simulink model "quadrotor_model_simulink_validation"  (R2018a)
settings: Solver=FixedStepDiscrete  StartTime=0.0  StopTime=40  FixedStep=Ts  RelTol=1e-3
PreLoadFcn:
  | % Quadrotor model
  | load('quadrotor_model.mat');
  | Ts = quadrotor_model.Ts;
  | d = 3;
InitFcn:
  | % Quadrotor model
  | load('quadrotor_model.mat');
  | Ts = quadrotor_model.Ts;
  | d = 3;
undefined symbols (not defined in the file): quadrotor_model
settings Model: Creator=silveira  LastModifiedBy=silveira
settings DebuggingCC: ReadBeforeWriteMsg=DisableAll  WriteAfterWriteMsg=DisableAll  WriteAfterReadMsg=DisableAll  MultiTaskDSMMsg=none
settings CodeAppCC: StateflowObjectComments=on

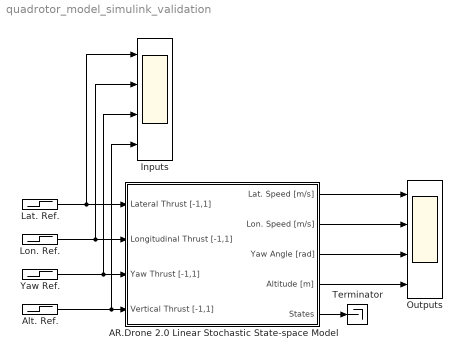
== system quadrotor_model_simulink_validation ==
  AR.Drone 2.0 Linear Stochastic State-space Model : Subsystem
  Alt. Ref. : Step  SampleTime=Ts
  Inputs : Scope  NumInputPorts=4
  Lat. Ref. : Step  SampleTime=Ts
  Lon. Ref. : Step  SampleTime=Ts
  Outputs : Scope  NumInputPorts=4
  Terminator : Terminator
  Yaw Ref. : Step  SampleTime=Ts
  wires:
  AR.Drone 2.0 Linear Stochastic State-space Model/5(States) -> Terminator/1
  Lat. Ref./1 -> Inputs/1, AR.Drone 2.0 Linear Stochastic State-space Model/1(Lateral Thrust [-1,1])
  Lon. Ref./1 -> Inputs/2, AR.Drone 2.0 Linear Stochastic State-space Model/2(Longitudinal Thrust [-1,1])
  Yaw Ref./1 -> Inputs/3, AR.Drone 2.0 Linear Stochastic State-space Model/3(Yaw Thrust [-1,1])
  Alt. Ref./1 -> Inputs/4, AR.Drone 2.0 Linear Stochastic State-space Model/4(Vertical Thrust [-1,1])
  AR.Drone 2.0 Linear Stochastic State-space Model/1(Lat. Speed [m/s]) -> Outputs/1
  AR.Drone 2.0 Linear Stochastic State-space Model/2(Lon. Speed [m/s]) -> Outputs/2
  AR.Drone 2.0 Linear Stochastic State-space Model/3(Yaw Angle [rad]) -> Outputs/3
  AR.Drone 2.0 Linear Stochastic State-space Model/4(Altitude [m]) -> Outputs/4

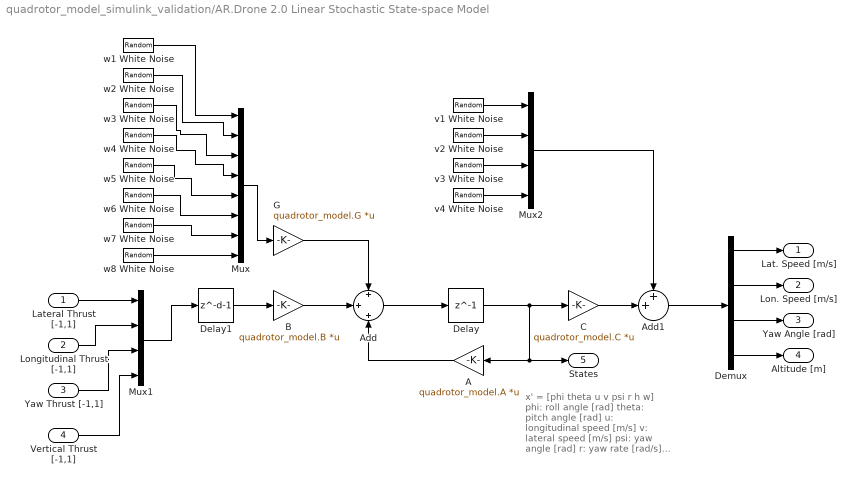
== system quadrotor_model_simulink_validation/AR.Drone 2.0 Linear Stochastic State-space Model ==
  note: x' = [phi theta u v psi r h w]
      |
      | phi: roll angle [rad]
      | theta: pitch angle [rad]
      | u: longitudinal speed [m/s]
      | v: lateral speed [m/s]
      | psi: yaw angle [rad]
      | r: yaw rate [rad/s]
      | h: altitude [m]
      | w: vertical speed [m/s]
  Lateral Thrust [-1,1] : Inport
  Longitudinal Thrust [-1,1] : Inport  Port=2
  Yaw Thrust [-1,1] : Inport  Port=3
  Vertical Thrust [-1,1] : Inport  Port=4
  A : Gain  Gain=quadrotor_model.A  Multiplication=Matrix(K*u)
  Add : Sum  Inputs=+|+|+
  Add1 : Sum  Inputs=++|
  B : Gain  Gain=quadrotor_model.B  Multiplication=Matrix(K*u)
  C : Gain  Gain=quadrotor_model.C  Multiplication=Matrix(K*u)
  Delay : Delay  DelayLength=1  SampleTime=Ts
  Delay1 : Delay  DelayLength=d-1  SampleTime=Ts
  Demux : Demux
  G : Gain  Gain=quadrotor_model.G  Multiplication=Matrix(K*u)
  Mux : Mux  Inputs=8
  Mux1 : Mux
  Mux2 : Mux
  v1 White Noise : RandomNumber  DisableCoverage=on  Variance=quadrotor_model.R(1,1)  Seed=8  SampleTime=Ts
  v2 White Noise : RandomNumber  DisableCoverage=on  Variance=quadrotor_model.R(2,2)  Seed=9  SampleTime=Ts
  v3 White Noise : RandomNumber  DisableCoverage=on  Variance=quadrotor_model.R(3,3)  Seed=10  SampleTime=Ts
  v4 White Noise : RandomNumber  DisableCoverage=on  Variance=quadrotor_model.R(4,4)  Seed=11  SampleTime=Ts
  w1 White Noise : RandomNumber  DisableCoverage=on  Variance=quadrotor_model.Q(1,1)  SampleTime=Ts
  w2 White Noise : RandomNumber  DisableCoverage=on  Variance=quadrotor_model.Q(2,2)  Seed=1  SampleTime=Ts
  w3 White Noise : RandomNumber  DisableCoverage=on  Variance=quadrotor_model.Q(3,3)  Seed=2  SampleTime=Ts
  w4 White Noise : RandomNumber  DisableCoverage=on  Variance=quadrotor_model.Q(4,4)  Seed=3  SampleTime=Ts
  w5 White Noise : RandomNumber  DisableCoverage=on  Variance=quadrotor_model.Q(5,5)  Seed=4  SampleTime=Ts
  w6 White Noise : RandomNumber  DisableCoverage=on  Variance=quadrotor_model.Q(6,6)  Seed=5  SampleTime=Ts
  w7 White Noise : RandomNumber  DisableCoverage=on  Variance=quadrotor_model.Q(7,7)  Seed=6  SampleTime=Ts
  w8 White Noise : RandomNumber  DisableCoverage=on  Variance=quadrotor_model.Q(8,8)  Seed=7  SampleTime=Ts
  Lat. Speed [m/s] : Outport
  Lon. Speed [m/s] : Outport  Port=2
  Yaw Angle [rad] : Outport  Port=3
  Altitude [m] : Outport  Port=4
  States : Outport  Port=5
  wires:
  A/1 -> Add/3
  w2 White Noise/1 -> Mux/2
  G/1 -> Add/1
  w1 White Noise/1 -> Mux/1
  Mux/1 -> G/1
  Add/1 -> Delay/1
  Delay/1 -> States/1, A/1, C/1
  C/1 -> Add1/2
  B/1 -> Add/2
  Delay1/1 -> B/1
  w3 White Noise/1 -> Mux/3
  w4 White Noise/1 -> Mux/4
  w5 White Noise/1 -> Mux/5
  w6 White Noise/1 -> Mux/6
  w7 White Noise/1 -> Mux/7
  w8 White Noise/1 -> Mux/8
  Mux1/1 -> Delay1/1
  Lateral Thrust [-1,1]/1 -> Mux1/1
  Longitudinal Thrust [-1,1]/1 -> Mux1/2
  Yaw Thrust [-1,1]/1 -> Mux1/3
  Vertical Thrust [-1,1]/1 -> Mux1/4
  Mux2/1 -> Add1/1
  v4 White Noise/1 -> Mux2/4
  v3 White Noise/1 -> Mux2/3
  v2 White Noise/1 -> Mux2/2
  v1 White Noise/1 -> Mux2/1
  Demux/4 -> Altitude [m]/1
  Demux/3 -> Yaw Angle [rad]/1
  Demux/2 -> Lon. Speed [m/s]/1
  Demux/1 -> Lat. Speed [m/s]/1
  Add1/1 -> Demux/1
